simulink model "sf_gfdemo"  (R2017b)
settings: Solver=ode45  StartTime=0.0  StopTime=10  MaxStep=.01  RelTol=1e-3  EnableMultiTasking=on
settings Model: FPTRunName=Active  ExtModeAutoUpdateStatusClock=off  Creator=The MathWorks, Inc.  LastModifiedBy=The MathWorks, Inc.
settings DataIOCC: LimitDataPoints=on  SaveFormat=Array
settings OptimizationCC: BooleanDataType=off  ExpressionDepthLimit=2147483647  InitFltsAndDblsToZero=on  EfficientMapNaN2IntZero=off  LifeSpan=inf
settings DebuggingCC: SaveWithParameterizedLinksMsg=none  UnderspecifiedInitializationDetection=Classic  MergeDetectMultiDrivingBlocksExec=none  SignalResolutionControl=TryResolveAllWithWarning  MultiTaskDSMMsg=warning  MultiTaskCondExecSysMsg=none  FcnCallInpInsideContextMsg=warning  StateNameClashWarn=warning  StrictBusMsg=None  SFUnexpectedBacktrackingDiag=warning  SFNoUnconditionalDefaultTransitionDiag=warning  SFExecutionAtInitializationDiag=none
settings HardwareCC: ProdBitPerPointer=32  ProdBitPerSizeT=32  ProdBitPerPtrDiffT=32  ProdLargestAtomicFloat=None  ProdIntDivRoundTo=Undefined  ProdEndianess=Unspecified  ProdWordSize=32  ProdHWDeviceType=32-bit Generic  TargetUnknown=on
settings ModelReferenceCC: PropagateSignalLabelsOutOfModel=off
settings SFSimCC: SimParseCustomCode=off
settings CodeAppCC: StateflowObjectComments=on
settings GRTTargetCC: TargetFcnLib=ansi_tfl_tmw.mat  TargetLangStandard=C89/C90 (ANSI)  GeneratePreprocessorConditionals=Disable all  CombineOutputUpdateFcns=off  GRTInterface=on
settings ConfigComp: CovMetricSettings=dcmtr  CovHtmlReporting=on  CovSaveCumulativeToWorkspaceVar=on  CovSaveSingleToWorkspaceVar=on  CovExternalEMLEnable=off  CovSFcnEnable=off

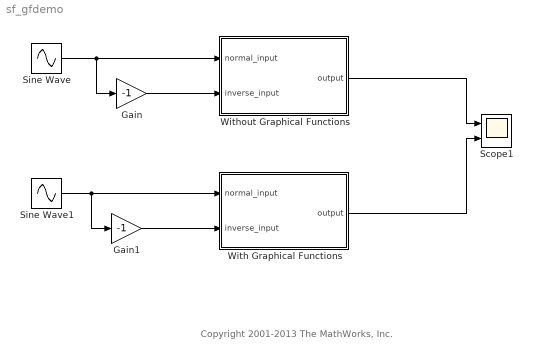
== system sf_gfdemo ==
  note: Copyright 2001-2013 The MathWorks, Inc.
  Gain : Gain  Gain=-1  SaturateOnIntegerOverflow=on  OutDataTypeStr=Inherit: Same as input  ParamDataTypeStr=Inherit: Same as input
  Gain1 : Gain  Gain=-1  SaturateOnIntegerOverflow=on  OutDataTypeStr=Inherit: Same as input  ParamDataTypeStr=Inherit: Same as input
  Scope1 : Scope  NumInputPorts=2
  Sine Wave : Sin  SampleTime=0
  Sine Wave1 : Sin  SampleTime=0
  With Graphical Functions : Stateflow chart  TreatAsAtomicUnit=on
  Without Graphical Functions : Stateflow chart  TreatAsAtomicUnit=on
  wires:
  Without Graphical Functions/1(output) -> Scope1/1
  With Graphical Functions/1(output) -> Scope1/2
  Sine Wave/1 -> Gain/1, Without Graphical Functions/1(normal_input)
  Gain/1 -> Without Graphical Functions/2(inverse_input)
  Sine Wave1/1 -> Gain1/1, With Graphical Functions/1(normal_input)
  Gain1/1 -> With Graphical Functions/2(inverse_input)

== stateflow chart sf_gfdemo/Without Graphical Functions ==
  state Normal
    (default) -> (junction 16)
    (junction 16) -> (junction 20) [order 1] : [normal_input >0.5]
    (junction 20) -> (junction 21) : {output = 0.5;}
    (junction 16) -> (junction 21) [order 2] : {output=normal_input;}
  state Inverse
    (default) -> (junction 17)
    (junction 17) -> (junction 18) [order 1] : [inverse_input > 0.5]
    (junction 17) -> (junction 19) [order 2] : {output=inverse_input;}
    (junction 18) -> (junction 19) : {output = 0.5;}
  (default) -> Normal
  Normal -> Normal [order 2]
  Normal -> Inverse [order 1] : [normal_input < 0]
  Inverse -> Normal [order 1] : [inverse_input<0]
  Inverse -> Inverse [order 2]
  data: output output double; normal_input input double; inverse_input input double

== stateflow chart sf_gfdemo/With Graphical Functions ==
  state Normal
    (default) -> (junction 16) : {set_output_data(normal_input);}
  state set_output_data(input) [function]
    (default) -> (junction 15)
    (junction 15) -> (junction 18) [order 1] : [input>.5]
    (junction 15) -> (junction 19) [order 2] : {output = input;}
    (junction 18) -> (junction 19) : {output = 0.5;}
  state Inverse
    (default) -> (junction 17) : {set_output_data(inverse_input);}
  (default) -> Normal
  Normal -> Normal [order 2]
  Inverse -> Normal [order 1] : [inverse_input<0]
  Normal -> Inverse [order 1] : [normal_input < 0]
  Inverse -> Inverse [order 2]
  data: input function_input double; output output double; normal_input input double; inverse_input input double
